simulink model "TTypeInverter"  (R2022b)
settings: Solver=ode15s  StartTime=0.0  StopTime=0.2  FixedStep=Ts  RelTol=1e-3
values from neighbouring files (symbols this model uses):
  C_c = 30*10^-6    (= 3e-05)    [TTypeInverterVals.m]
  den = abs(G_pr_r_z.Denominator{1,1})    [TTypeInverterVals.m]
  den15 = abs(G_pr_r_15_z.Denominator{1,1})    [TTypeInverterVals.m]
  den21 = abs(G_pr_r_21_z.Denominator{1,1})    [TTypeInverterVals.m]
  den5 = abs(G_pr_r_5_z.Denominator{1,1})    [TTypeInverterVals.m]
  den7 = abs(G_pr_r_7_z.Denominator{1,1})    [TTypeInverterVals.m]
  f_o = 50    [TTypeInverterVals.m]
  G_diff_z = c2d(G_diff_s,Ts,opt)    [ControllerDesign.m]    (also in TTypeInverterVals.m = c2d(G_diff_s,Ts,'foh'))
  Kc = 0.35    [ControllerDesign.m]    (also in TTypeInverterVals.m = 2.5)
  Klim = 5    [TTypeInverterVals.m]
  Kp = 1/mag    [ControllerDesign.m]    (also in TTypeInverterVals.m = 0.9444)
  Kr = []    [ControllerDesign.m]    (also in TTypeInverterVals.m = 3141.59265359)
  KT = []    [ControllerDesign.m]
  num = abs(G_pr_r_z.Numerator{1,1})    [TTypeInverterVals.m]
  num15 = abs(G_pr_r_15_z.Numerator{1,1})    [TTypeInverterVals.m]
  num21 = abs(G_pr_r_21_z.Numerator{1,1})    [TTypeInverterVals.m]
  num5 = abs(G_pr_r_5_z.Numerator{1,1})    [TTypeInverterVals.m]
  num7 = abs(G_pr_r_7_z.Numerator{1,1})    [TTypeInverterVals.m]
  omega_o = fo*2*pi    (= 314.159265359)    [ControllerDesign.m]    (also in TTypeInverterVals.m)
  omega_w = []    [ControllerDesign.m]    (also in TTypeInverterVals.m = 0.628318530718)
  pr_sat_val = ceil(3*io_nom)    [TTypeInverterVals.m]
  R = [R_iL 0 ... (first row only)    [TTypeInverterVals.m]
  R_l_20p = Vout^2/P_lin_20p    (= 10.58)    [TTypeInverterVals.m]
  R_l_80p = Vout^2/P_lin_80p    (= 2.645)    [TTypeInverterVals.m]
  R_l_nl = Vout^2/P_lin    (= 3.11176470588)    [TTypeInverterVals.m]
  R_Lc = 5.6e-3    (= 0.0056)    [TTypeInverterVals.m]
  R_nl_load = Uc^2/(0.66*S_tot)    (= 14.9121893939)    [TTypeInverterVals.m]
  R_nl_s = 0.04*Vout^2/S_tot    (= 0.2645)    [TTypeInverterVals.m]
  Tcomp = T_sw/8    (= 5.20833333333e-06)    [TTypeInverterVals.m]
  Ts = 1/(fs)    (= 2.08333333333e-05)    [ControllerDesign.m]    (also in KalmanFilter.m; TTypeInverterVals.m = 1.04160003681e-05)
  VDC = 800    [TTypeInverterVals.m]
  Vout_amp = 230*sqrt(2)    [TTypeInverterVals.m]
undefined symbols (not defined in the file or in its folder): a0, a1, b0, b1, G_ll_z, Ki, Kpc, kv, UKF_data
libraries: ee_lib x29, nesl_utility x14, fl_lib x10, dspstat3 x5, spsTriangleGeneratorLib x2, spsRMSLib x1, spsTHDLib x1, spspowerguiLib x1
(part 2 of 2)

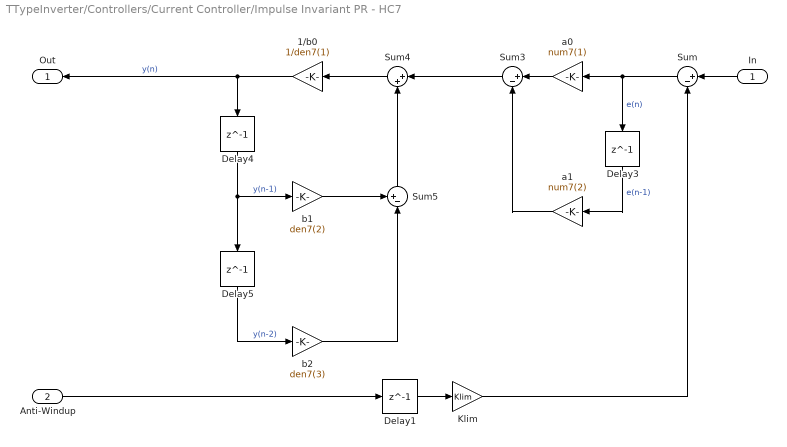
== system TTypeInverter/Controllers/Current Controller/Impulse Invariant PR - HC7 ==
  In : Inport
  Anti-Windup : Inport  Port=2
  1/b0 : Gain  Gain=1/den7(1)
  Delay{1,3..5} (4 alike) : Delay  DelayLength=1  SampleTime=Ts
  Klim : Gain  Gain=Klim
  Sum : Sum  Inputs=|+-
  Sum3 : Sum  Inputs=|+-
  Sum4 : Sum  Inputs=|++
  Sum5 : Sum  Inputs=+-|
  a0 : Gain  Gain=num7(1)
  a1 : Gain  Gain=num7(2)
  b1 : Gain  Gain=den7(2)
  b2 : Gain  Gain=den7(3)
  Out : Outport
  wires:
  Delay3/1 -> a1/1  "e(n-1)"
  Delay5/1 -> b2/1  "y(n-2)"
  1/b0/1 -> Out/1, Delay4/1  "y(n)"
  Sum3/1 -> Sum4/1
  Sum4/1 -> 1/b0/1
  b2/1 -> Sum5/2
  Sum5/1 -> Sum4/2
  b1/1 -> Sum5/1
  Delay4/1 -> Delay5/1, b1/1  "y(n-1)"
  a0/1 -> Sum3/1
  a1/1 -> Sum3/2
  Klim/1 -> Sum/2
  Anti-Windup/1 -> Delay1/1
  Delay1/1 -> Klim/1
  Sum/1 -> a0/1, Delay3/1  "e(n)"
  In/1 -> Sum/1

== system TTypeInverter/Controllers/Current Controller/Lead-Lag ==
  In : Inport
  Delay : Delay  DelayLength=1  SampleTime=Ts
  Delay1 : Delay  DelayLength=1  SampleTime=Ts
  Gain : Gain  Gain=C_c
  Gain1 : Gain
  Sum : Sum  Inputs=|++
  Sum1 : Sum  Inputs=|++
  a0 : Gain  Gain=a0
  a1 : Gain  Gain=a1
  b0 : Gain  Gain=b0
  b1 : Gain  Gain=b1
  Out : Outport
  wires:
  Gain1/1 -> Out/1
  Gain/1 -> Gain1/1
  In/1 -> Delay/1, a0/1  "e(n)"
  a0/1 -> Sum/1
  Delay/1 -> a1/1  "e(n-1)"
  a1/1 -> Sum/2
  Sum/1 -> Sum1/1
  Delay1/1 -> b1/1  "y(n-1)"
  b1/1 -> Sum1/2
  Sum1/1 -> b0/1
  b0/1 -> Delay1/1, Gain/1  "y(n)"

== system TTypeInverter/Controllers/Current Controller/PI Controller ==
  In : Inport
  Delay : Delay  DelayLength=1  SampleTime=Ts
  Gain1 : Gain  Gain=Kpc
  Gain2 : Gain  Gain=Ki
  Gain3 : Gain  Gain=Ts
  Sum2 : Sum  Inputs=++|
  Sum3 : Sum  Inputs=|++
  Out : Outport
  wires:
  Gain1/1 -> Sum2/1
  Gain2/1 -> Gain3/1
  Sum3/1 -> Sum2/2, Delay/1
  Gain3/1 -> Sum3/1
  Delay/1 -> Sum3/2
  In/1 -> Gain1/1, Gain2/1
  Sum2/1 -> Out/1

== system TTypeInverter/Controllers/Voltage Controller/Fifth Harmonic ==
  In : Inport
  Anti-Windup : Inport  Port=2
  1/b0 : Gain  Gain=1/(KT(3)*KT(3)+2*omega_w(3)*KT(3)+5*5*omega_o*omega_o)
  Delay1 : Delay  DelayLength=1  SampleTime=Ts
  Delay3 : Delay  SampleTime=Ts
  Delay4 : Delay  DelayLength=1  SampleTime=Ts
  Delay5 : Delay  DelayLength=1  SampleTime=Ts
  Klim : Gain  Gain=Klim
  Sum : Sum  Inputs=|+-
  Sum3 : Sum  Inputs=|+-
  Sum4 : Sum  Inputs=|++
  Sum5 : Sum  Inputs=+-|
  a1 : Gain  Gain=2*Kr(3)*KT(3)*omega_w(3)
  b1 : Gain  Gain=2*KT(3)*KT(3)-2*5*5*omega_o*omega_o
  b2 : Gain  Gain=KT(3)*KT(3)+2*omega_w(3)*KT(3)-5*5*omega_o*omega_o
  Out : Outport
  wires:
  Delay3/1 -> Sum3/2  "e(n-2)"
  Delay5/1 -> b2/1  "y(n-2)"
  Klim/1 -> Sum/2
  1/b0/1 -> Out/1, Delay4/1  "y(n)"
  a1/1 -> Sum4/1
  Sum4/1 -> 1/b0/1
  Sum3/1 -> a1/1
  b2/1 -> Sum5/2
  Sum5/1 -> Sum4/2
  Sum/1 -> Sum3/1, Delay3/1  "e(n)"
  b1/1 -> Sum5/1
  Delay4/1 -> Delay5/1, b1/1  "y(n-1)"
  In/1 -> Sum/1
  Delay1/1 -> Klim/1
  Anti-Windup/1 -> Delay1/1

== system TTypeInverter/Controllers/Voltage Controller/Fundamental ==
  In : Inport
  Anti-Windup : Inport  Port=2
  1/b0 : Gain  Gain=1/(KT(1)*KT(1)+2*omega_w(1)*KT(1)+omega_o*omega_o)
  Delay1 : Delay  DelayLength=1  SampleTime=Ts
  Delay3 : Delay  SampleTime=Ts
  Delay4 : Delay  DelayLength=1  SampleTime=Ts
  Delay5 : Delay  DelayLength=1  SampleTime=Ts
  Klim : Gain  Gain=Klim
  Sum : Sum  Inputs=|+-
  Sum3 : Sum  Inputs=|+-
  Sum4 : Sum  Inputs=|++
  Sum5 : Sum  Inputs=+-|
  a1 : Gain  Gain=2*Kr(1)*KT(1)*omega_w(1)
  b1 : Gain  Gain=2*KT(1)*KT(1)-2*omega_o*omega_o
  b2 : Gain  Gain=KT(1)*KT(1)+2*omega_w(1)*KT(1)-omega_o*omega_o
  Out : Outport
  wires:
  Delay3/1 -> Sum3/2  "e(n-2)"
  Delay5/1 -> b2/1  "y(n-2)"
  Klim/1 -> Sum/2
  1/b0/1 -> Out/1, Delay4/1  "y(n)"
  a1/1 -> Sum4/1
  Sum4/1 -> 1/b0/1
  Sum3/1 -> a1/1
  b2/1 -> Sum5/2
  Sum5/1 -> Sum4/2
  Sum/1 -> Sum3/1, Delay3/1  "e(n)"
  b1/1 -> Sum5/1
  Delay4/1 -> Delay5/1, b1/1  "y(n-1)"
  In/1 -> Sum/1
  Delay1/1 -> Klim/1
  Anti-Windup/1 -> Delay1/1

== system TTypeInverter/Controllers/Voltage Controller/Impulse Invariant PR - Fundamental ==
  e_out : Inport
  Anti-Windup : Inport  Port=2
  1/b0 : Gain  Gain=1/den(1)
  Delay{1,3..5} (4 alike) : Delay  DelayLength=1  SampleTime=Ts
  Klim : Gain  Gain=Klim
  Sum : Sum  Inputs=|+-
  Sum3 : Sum  Inputs=|+-
  Sum4 : Sum  Inputs=|++
  Sum5 : Sum  Inputs=+-|
  a0 : Gain  Gain=num(1)
  a1 : Gain  Gain=num(2)
  b1 : Gain  Gain=den(2)
  b2 : Gain  Gain=den(3)
  Out : Outport
  wires:
  Delay3/1 -> a1/1  "e(n-1)"
  Delay5/1 -> b2/1  "y(n-2)"
  Klim/1 -> Sum/2
  1/b0/1 -> Out/1, Delay4/1  "y(n)"
  Sum3/1 -> Sum4/1
  Sum4/1 -> 1/b0/1
  b2/1 -> Sum5/2
  Sum5/1 -> Sum4/2
  Sum/1 -> a0/1, Delay3/1  "e(n)"
  b1/1 -> Sum5/1
  Delay4/1 -> Delay5/1, b1/1  "y(n-1)"
  e_out/1 -> Sum/1
  Delay1/1 -> Klim/1
  Anti-Windup/1 -> Delay1/1
  a0/1 -> Sum3/1
  a1/1 -> Sum3/2

== system TTypeInverter/Controllers/Voltage Controller/Non-prewarped Tustin-based PR ==
  In1 : Inport
  1/(Ts*Ts*omega_0*omega_0+4*Ts*omega_w+4) : Gain  Gain=1/(Ts*Ts*omega_o*omega_o+4*Ts*omega_w(1)+4)
  2*Ts*Ts*omega_0*omega_0 : Gain  Gain=2*Ts*Ts*omega_o*omega_o-8
  4*Ts*omega_w : Gain  Gain=4*Ts*omega_w(1)
  4*Ts*omega_w! : Gain  Gain=4*Ts*omega_w(1)
  Add1 : Sum
  Delay3 : Delay  SampleTime=Ts
  Delay4 : Delay  DelayLength=1  SampleTime=Ts
  Delay5 : Delay  DelayLength=1  SampleTime=Ts
  Multiply2 : Gain  Gain=Kp
  Multiply3 : Gain  Gain=Kr(1)
  Saturation : Saturate  UpperLimit=pr_sat_val  LowerLimit=-pr_sat_val
  Sum3 : Sum  Inputs=|+-
  Sum4 : Sum  Inputs=|+-
  Sum5 : Sum  Inputs=++|
  Ts*Ts*omega_0*omega_0-4*Ts*omega_w : Gain  Gain=Ts*Ts*omega_o*omega_o-4*Ts*omega_w(1)+4
  Out1 : Outport
  wires:
  Multiply2/1 -> Add1/1
  Delay4/1 -> Delay5/1, 2*Ts*Ts*omega_0*omega_0/1
  Delay5/1 -> Ts*Ts*omega_0*omega_0-4*Ts*omega_w/1
  Multiply3/1 -> Delay3/1, 4*Ts*omega_w/1
  Delay3/1 -> 4*Ts*omega_w!/1
  Sum3/1 -> Sum4/1
  In1/1 -> Multiply3/1, Multiply2/1
  4*Ts*omega_w/1 -> Sum3/1
  Saturation/1 -> Out1/1
  Ts*Ts*omega_0*omega_0-4*Ts*omega_w/1 -> Sum5/2
  4*Ts*omega_w!/1 -> Sum3/2
  Sum5/1 -> Sum4/2
  Sum4/1 -> 1/(Ts*Ts*omega_0*omega_0+4*Ts*omega_w+4)/1
  Add1/1 -> Saturation/1
  1/(Ts*Ts*omega_0*omega_0+4*Ts*omega_w+4)/1 -> Add1/2, Delay4/1
  2*Ts*Ts*omega_0*omega_0/1 -> Sum5/1

== system TTypeInverter/Controllers/Voltage Controller/Seventh Harmonic ==
  In : Inport
  Anti-Windup : Inport  Port=2
  1/b0 : Gain  Gain=1/(KT(4)*KT(4)+2*omega_w(4)*KT(4)+7*omega_o*omega_o)
  Delay1 : Delay  DelayLength=1  SampleTime=Ts
  Delay3 : Delay  SampleTime=Ts
  Delay4 : Delay  DelayLength=1  SampleTime=Ts
  Delay5 : Delay  DelayLength=1  SampleTime=Ts
  Klim : Gain  Gain=Klim
  Sum : Sum  Inputs=|+-
  Sum3 : Sum  Inputs=|+-
  Sum4 : Sum  Inputs=|++
  Sum5 : Sum  Inputs=+-|
  a1 : Gain  Gain=2*Kr(4)*KT(4)*omega_w(4)
  b1 : Gain  Gain=2*KT(4)*KT(4)-2*7*omega_o*omega_o
  b2 : Gain  Gain=KT(4)*KT(4)+2*omega_w(4)*KT(4)-7*omega_o*omega_o
  Out : Outport
  wires:
  Delay3/1 -> Sum3/2  "e(n-2)"
  Delay5/1 -> b2/1  "y(n-2)"
  Klim/1 -> Sum/2
  1/b0/1 -> Out/1, Delay4/1  "y(n)"
  a1/1 -> Sum4/1
  Sum4/1 -> 1/b0/1
  Sum3/1 -> a1/1
  b2/1 -> Sum5/2
  Sum5/1 -> Sum4/2
  Sum/1 -> Sum3/1, Delay3/1  "e(n)"
  b1/1 -> Sum5/1
  Delay4/1 -> Delay5/1, b1/1  "y(n-1)"
  In/1 -> Sum/1
  Delay1/1 -> Klim/1
  Anti-Windup/1 -> Delay1/1

== system TTypeInverter/Controllers/Voltage Controller/Third Harmonic ==
  In : Inport
  Anti-Windup : Inport  Port=2
  1/b0 : Gain  Gain=1/(KT(2)*KT(2)+2*omega_w(2)*KT(2)+3*3*omega_o*omega_o)
  Delay1 : Delay  DelayLength=1  SampleTime=Ts
  Delay3 : Delay  SampleTime=Ts
  Delay4 : Delay  DelayLength=1  SampleTime=Ts
  Delay5 : Delay  DelayLength=1  SampleTime=Ts
  Klim : Gain  Gain=Klim
  Sum : Sum  Inputs=|+-
  Sum3 : Sum  Inputs=|+-
  Sum4 : Sum  Inputs=|++
  Sum5 : Sum  Inputs=+-|
  a1 : Gain  Gain=2*Kr(2)*KT(2)*omega_w(2)
  b1 : Gain  Gain=2*KT(2)*KT(2)-2*3*3*omega_o*omega_o
  b2 : Gain  Gain=KT(2)*KT(2)+2*omega_w(2)*KT(2)-3*3*omega_o*omega_o
  Out : Outport
  wires:
  Delay3/1 -> Sum3/2  "e(n-2)"
  Delay5/1 -> b2/1  "y(n-2)"
  Klim/1 -> Sum/2
  1/b0/1 -> Out/1, Delay4/1  "y(n)"
  a1/1 -> Sum4/1
  Sum4/1 -> 1/b0/1
  Sum3/1 -> a1/1
  b2/1 -> Sum5/2
  Sum5/1 -> Sum4/2
  Sum/1 -> Sum3/1, Delay3/1  "e(n)"
  b1/1 -> Sum5/1
  Delay4/1 -> Delay5/1, b1/1  "y(n-1)"
  In/1 -> Sum/1
  Delay1/1 -> Klim/1
  Anti-Windup/1 -> Delay1/1

== matlab function TTypeInverter/Kalman Filter - Unscented/Unscented Kalman Filter/Predict Step ==
  data: yhat_minus output; xhat_k input; P_k input; P_minus output; u_k input; xhat_minus output; UKF_struct parameter
function [yhat_minus, P_minus, xhat_minus] = fcn(xhat_k, P_k, u_k, UKF_struct)

% For testing with and without including the mean value
calc = 'WithoutMean';

if strcmp(calc,'WithoutMean')
    n = 2*UKF_struct.n;
    w = 1/(2*(UKF_struct.n+UKF_struct.kappa))*ones(n,1);
elseif strcmp(calc, 'WithMean')
    n = 2*UKF_struct.n+1;
    w = [0.5*ones(length(xhat_k),1); UKF_struct.kappa; 0.5*ones(length(xhat_k),1)]/(UKF_struct.n+UKF_struct.kappa);
else
    disp('Calculation type error in Unscented Kalman filter')
end


% Initialize variables
x_sigma = zeros(length(xhat_k), n);
xhat_sigma = zeros(length(xhat_k), n);
yhat_minus = zeros(height(UKF_struct.C), 1);


% 1) Calculate x-sigma points (xhat sigmas)
P_k_sqrt = real(sqrtm((UKF_struct.n+UKF_struct.kappa)*P_k));
for i = 1:length(xhat_k)
    x_sigma(:,i) = xhat_k(:) + P_k_sqrt(:,i);
    if strcmp(calc,'WithoutMean')
        x_sigma(:,i+UKF_struct.n) = xhat_k(:) - P_k_sqrt(:,i);
    elseif strcmp(calc,'WithMean')
        x_sigma(:,i+UKF_struct.n+1) = xhat_k(:) - P_k_sqrt(:,i);
        x_sigma(:,UKF_struct.n+1) = xhat_k(:);
    end
end


% 2) Calculate y-sigma points (xhat_minus sigmas)
for i = 1:n
    xhat_sigma(:,i) = [x_sigma(1,i) + UKF_struct.Ts*( ((2.2737*abs(x_sigma(1,i)))^1.9167+44052.86)/3.9813 * (u_k(1) - x_sigma(1,i)*UKF_struct.RLc - x_sigma(3,i)*UKF_struct.RCc - x_sigma(2,i)) ); ...
                       x_sigma(2,i) + UKF_struct.Ts*x_sigma(3,i)/UKF_struct.Cc; ...
                       x_sigma(1,i) - u_k(2)];

                       % Calculate ic from next iL - io
                       % x_sigma(1,i) + UKF_struct.Ts*( ((2.2737*abs(x_sigma(1,i)))^1.9167+44052.86)/3.9813 * (u_k(1) - x_sigma(1,i)*UKF_struct.RLc - x_sigma(3,i)*UKF_struct.RCc - x_sigma(2,i)) ) - u_k(2)];
                       
                       % Calculate ic by taking diL and calculating dio
                       %x_sigma(3,i) + UKF_struct.Ts*UKF_struct.Cc*(x_sigma(1,i)+(1/UKF_struct.Lg)*(x_sigma(2,i) - u_k(2)*UKF_struct.RLg + x_sigma(3,i)*UKF_struct.RCc) )];
                       
                       % Calculate ic by calculating both diL and dio
                       %x_sigma(3,i) + UKF_struct.Ts*UKF_struct.Cc*( ((2.2737*abs(x_sigma(1,i)))^1.9167+44052.86)/3.9813 * (u_k(1) - x_sigma(1,i)*UKF_struct.RLc - x_sigma(3,i)*UKF_struct.RCc - x_sigma(2,i)) ...
                       %- (1/UKF_struct.Lg)*(x_sigma(2,i) - u_k(2)*UKF_struct.RLg + x_sigma(3,i)*UKF_struct.RCc) )];
end


% 3) Predict states and outputs
xhat_minus = xhat_sigma*w;

yhat_minus(1) = xhat_minus(1);
yhat_minus(2) = xhat_minus(2) + xhat_minus(3)*UKF_struct.RCc;


% 4) Predict error covariance
P_minus = (xhat_sigma-xhat_minus)*diag(w)*(xhat_sigma-xhat_minus)' + UKF_struct.Q;

== matlab function TTypeInverter/Controllers/Current Controller/Variable Gain ==
  data: iL input; e_out output; e_in input
function e_out = fcn(iL, e_in)

% Create gain that somewhat follows the inductance graph (by linearization)
if abs(iL)<=218
    e_out = e_in - e_in*abs(iL)*1/218;
else
    e_out = 0;
end

== matlab function TTypeInverter/Kalman Filter - Unscented/Unscented Kalman Filter/Update Step ==
  data: y input; yhat_minus input; P_minus input; xhat_minus input; yhat output; xhat output; UKF_struct parameter; P output
function [yhat, xhat, P] = fcn(y, yhat_minus, P_minus, xhat_minus, UKF_struct)


% 1) Calculate Kalman gain
Lk = ( P_minus*(UKF_struct.C') ) * inv( UKF_struct.C*P_minus*(UKF_struct.C') + UKF_struct.R );


% 2) Update predictions
xhat = xhat_minus + Lk*(y-yhat_minus);
yhat = UKF_struct.C * xhat;


% 3) Update error covariance
P = (eye(length(P_minus)) - Lk*UKF_struct.C)*P_minus;
